simulink model "PSO_PID_Frecuencia"  (R2025a)
settings: Solver=FixedStepAuto  StartTime=0.0  StopTime=19  FixedStep=0.01  RelTol=1e-3
undefined symbols (not defined in the file or in its folder): CR, Kc_sim, LF, Td_sim, Ti_sim
libraries: instrumentseriallib x3
settings Model: Creator=jorge  LastModifiedBy=sergio2416

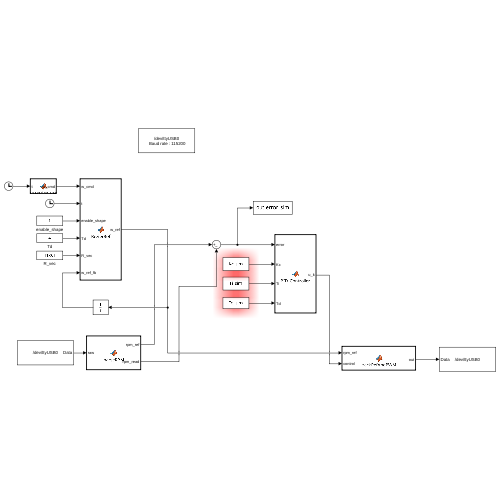
[thumbnail: Simulink's stored preview of the top-level diagram]
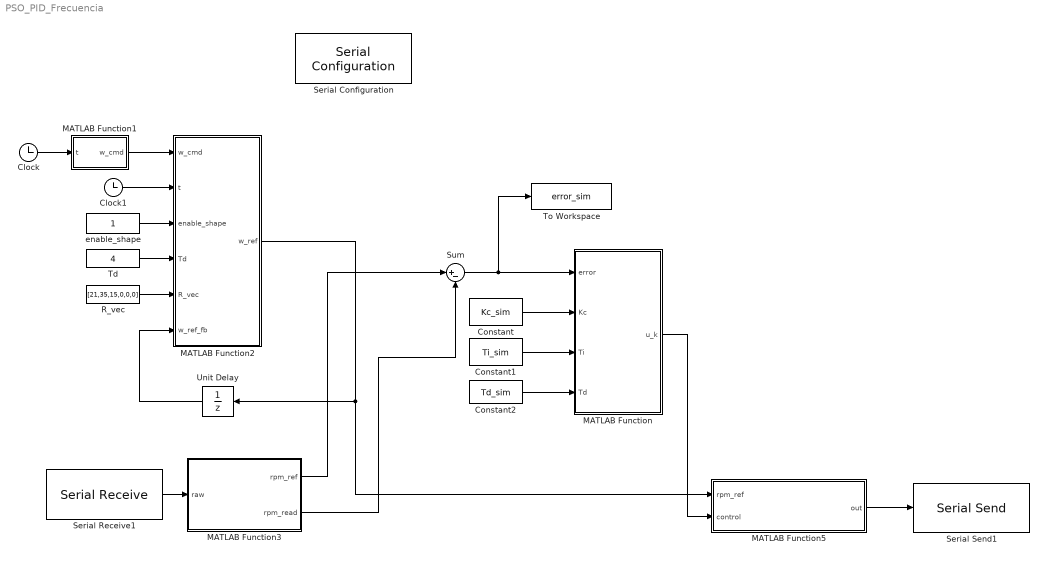
== system PSO_PID_Frecuencia ==
  Clock : Clock
  Clock1 : Clock
  Constant : Constant  Value=Kc_sim
  Constant1 : Constant  Value=Ti_sim
  Constant2 : Constant  Value=Td_sim
  MATLAB Function : MATLAB Function  TreatAsAtomicUnit=on
  MATLAB Function1 : MATLAB Function  TreatAsAtomicUnit=on
  MATLAB Function2 : MATLAB Function  TreatAsAtomicUnit=on
  MATLAB Function3 : MATLAB Function  TreatAsAtomicUnit=on
  MATLAB Function5 : MATLAB Function  TreatAsAtomicUnit=on
  R_vec : Constant  Value=[21,35,15,0,0,0]  SampleTime=-1
  Serial Configuration : instrumentseriallib/Serial Configuration  Priority=-200000  PortSel=/dev/ttyUSB0  Port=/dev/ttyUSB0  ComPort=/dev/ttyUSB0  BaudRate=115200  DataBits=8  Parity=none  StopBits=1  ByteOrder=little-endian  FlowControl=none  Timeout=10  SimulateUsing=Interpreted execution  BlockInModel=on  aMode=1
  Serial Receive1 : instrumentseriallib/Serial Receive  Priority=1  PortSel=/dev/ttyUSB0  Port=/dev/ttyUSB0  ComPort=/dev/ttyUSB0  DataType=int16  SaveDataType=uint8  ToggleHeader=off  Header=[]  ToggleDataSize=on  DataSize=[2 1]  ToggleTerminator=off  Terminator=CR/LF ('\r\n')  CustomTerminator=[]  InputFormat=Column major  EnableBlockingMode=on  ActionDataUnavailable=Output last received value  ActionWhenDataUnavailable=Output last received value  CustomValue=0  SampleTime=0.01  SimulateUsing=Interpreted execution  BlockInModel=on  aMode=1  LibraryInUse=instrumentlib
  Serial Send1 : instrumentseriallib/Serial Send  Priority=1  PortSel=/dev/ttyUSB0  Port=/dev/ttyUSB0  ComPort=/dev/ttyUSB0  Header=[]  Terminator=<none>  CustomTerminator=[]  EnableBlockingMode=off  SimulateUsing=Interpreted execution  BlockInModel=on  aMode=1
  Sum : Sum  Inputs=|+-
  Td : Constant  Value=4  SampleTime=-1
  To Workspace : ToWorkspace  VariableName=error_sim  SaveFormat=Timeseries  SampleTime=-1
  Unit Delay : UnitDelay  SampleTime=-1  HasFrameUpgradeWarning=on
  enable_shape : Constant  SampleTime=-1
  wires:
  Sum/1 -> To Workspace/1, MATLAB Function/1(error)
  Constant/1 -> MATLAB Function/2(Kc)
  Constant1/1 -> MATLAB Function/3(Ti)
  Constant2/1 -> MATLAB Function/4(Td)
  Clock/1 -> MATLAB Function1/1(t)
  Clock1/1 -> MATLAB Function2/2(t)
  enable_shape/1 -> MATLAB Function2/3(enable_shape)
  Td/1 -> MATLAB Function2/4(Td)
  MATLAB Function1/1(w_cmd) -> MATLAB Function2/1(w_cmd)
  R_vec/1 -> MATLAB Function2/5(R_vec)
  Unit Delay/1 -> MATLAB Function2/6(w_ref_fb)
  MATLAB Function5/1(out) -> Serial Send1/1
  Serial Receive1/1 -> MATLAB Function3/1(raw)
  MATLAB Function3/2(rpm_read) -> Sum/2
  MATLAB Function3/1(rpm_ref) -> Sum/1
  MATLAB Function2/1(w_ref) -> MATLAB Function5/1(rpm_ref), Unit Delay/1
  MATLAB Function/1(u_k) -> MATLAB Function5/2(control)

== matlab function PSO_PID_Frecuencia/MATLAB Function1 ==
  data: t input; w_cmd output
function w_cmd = Generador_Perfil(t)
    % Genera la señal escalón para alimentar al suavizador Bezier
    % Secuencia: 540 -> 1160 -> 800
    
    % --- CONFIGURACIÓN DE TIEMPOS ---
    % Td es 4 segundos. Dejamos un margen para que se estabilice.
    t_inicio = 1;   % Tiempo para el primer cambio (540 -> 1160)
    t_bajada = 10;  % Tiempo para el segundo cambio (1160 -> 800)
    
    % --- LÓGICA DE COMANDO ---
    if t < t_inicio
        % Estado inicial
        w_cmd = 600;
        
    elseif t >= t_inicio && t < t_bajada
        % Primer escalón: Subida
        w_cmd = 1160;
        
    else
        % Segundo escalón: Bajada
        w_cmd = 800;
    end
end

== matlab function PSO_PID_Frecuencia/MATLAB Function2 ==
  settings: updateMethod=DISCRETE
  data: w_cmd input; t input; w_ref output; enable_shape input; Td input; R_vec input; w_ref_fb input
function w_ref = BezierRef(w_cmd, t, enable_shape, Td, R_vec, w_ref_fb)
% =================================================================
% VERSIÓN 6 (Corrección de arranque en cero)
% =================================================================
%
% Entradas:
%   w_cmd     : setpoint deseado (de la GUI)
%   t         : tiempo absoluto (Clock)
%   enable_shape : 1 = perfilar, 0 = paso directo
%   Td        : duración de la transición [s]
%   R_vec     : [r1..r6] coeficientes del polinomio
%   w_ref_fb  : w_ref anterior (feedback vía Memory/Unit Delay)
%
% Salida:
%   w_ref     : referencia suavizada

% --- estados persistentes ---
persistent w0 wf t0 last_cmd is_initialized

% --- Lógica de inicialización en el primer paso de ejecución ---
if isempty(is_initialized) || t == 0 % Se reinicia si el tiempo es 0
    is_initialized = true; 
    
    % --- CORRECCIÓN AQUÍ ---
    % Antes decía: w0 = w_ref_fb; (Esto tomaba el 0 del Unit Delay)
    % Ahora dice:
    w0 = w_cmd;  % Forzamos a que el punto de partida sea el comando actual (540)
    wf = w_cmd;
    
    t0 = t;
    last_cmd = w_cmd;
end

% --- FIX 1: Detecta cambio de comando con tolerancia ---
if abs(w_cmd - last_cmd) > 1e-6
    % AQUÍ SÍ usamos w_ref_fb, porque queremos una curva suave desde
    % donde nos quedamos anteriormente.
    w0 = w_ref_fb;
    wf = w_cmd;
    t0 = t;
    last_cmd = w_cmd;
end

% Paso directo si está desactivado
if enable_shape == 0 || Td <= 0
    w_ref = w_cmd;
    w0 = w_cmd; 
    wf = w_cmd;
    last_cmd = w_cmd;
    return
end

% Progreso normalizado en [0,1]
s = (t - t0) / Td;

if s <= 0
    alpha = 0;
elseif s >= 1
    alpha = 1;
else
    % Bezier polinómico
    if numel(R_vec) < 6
        alpha = s; % Fallback a rampa lineal
    else
        r1 = R_vec(1); r2 = R_vec(2); r3 = R_vec(3);
        r4 = R_vec(4); r5 = R_vec(5); r6 = R_vec(6);
        
        % Validación de coeficientes
        if abs((r1 - r2 + r3 - r4 + r5 - r6) - 1.0) > 1e-3
            alpha = s^5;
        else
            alpha = (s.^5).*(r1 - r2*s + r3*s.^2 - r4*s.^3 + r5*s.^4 - r6*s.^5);
        end
    end
    
    % Clampeo por seguridad numérica
    if alpha < 0, alpha = 0; end
    if alpha > 1, alpha = 1; end
end

% Interpolación entre w0 y wf
w_ref = w0 + alpha*(wf - w0);
end

== matlab function PSO_PID_Frecuencia/MATLAB Function3 ==
  data: rpm_ref output; rpm_read output; raw input
function [rpm_ref, rpm_read] = parseRPM(raw)
%#codegen
% raw: 1x2 uint16 vector received from ESP32
% rpm_read: measured RPM from encoder
% rpm_ref:  reference RPM echoed back from ESP32

rpm_read = double(raw(2));   % first  uint16 from ESP32
rpm_ref  = double(raw(1));   % second uint16 from ESP32
end

== matlab function PSO_PID_Frecuencia/MATLAB Function5 ==
  data: rpm_ref input; control input; out output
function out = packRefAndPWM(rpm_ref, control)
% Esta función ahora empaqueta [rpm_ref, frequency_hz]
% El 'control_signal' (antes 'voltage') viene de 0-60 desde el "Knob".

% --- 1. Escalado lineal ---
% Frecuencia (0-60 Hz)
target_freq = control;

% --- 2. Empaquetado ---
% Convierte ambos valores a uint16 para enviar por UART
freq_u16 = uint16(target_freq);
rpm_ref_u16 = uint16(rpm_ref);

% El ESP32 espera recibir: [rpm_ref, frecuencia_en_hz]
out = uint16([rpm_ref_u16, freq_u16]);

end

== matlab function PSO_PID_Frecuencia/MATLAB Function ==
  data: error input; u_k output; Kc input; Ti input; Td input
function u_k = PID_Controller(error, Kc, Ti, Td)
    % ENTRADAS (Puertos en Simulink):
    %   error: Señal de error (Referencia - Salida)
    %   Kc, Ti, Td: Parámetros que vienen del Workspace (vía bloques Constant)
    
    % PARÁMETROS FIJOS (Ajusta si tu muestreo es distinto)
    Ts_s = 0.01;  % Tiempo de muestreo
    N = 100;      % Coeficiente del filtro derivativo

    % VARIABLES DE ESTADO (Persistentes)
    persistent error_prev integral_prev derivative_prev

    % INICIALIZACIÓN (Se ejecuta al inicio de CADA simulación 'sim')
    if isempty(error_prev)
        error_prev = 0.0;
        integral_prev = 0.0; % Ojo: Si tu salida debe empezar en 20, considera inicializar esto distinto
        derivative_prev = 0.0;
    end

    % --- 1. Proporcional ---
    p_k = Kc * error;

    % --- 2. Integral ---
    % Protección para Ti muy pequeño
    if Ti < 1e-6
        i_k = 0;
    else
        % Integración Euler
        i_k = integral_prev + (Kc * Ts_s / Ti) * error;
    end

    % --- 3. Derivativo ---
    c1 = 1.0 / (1.0 + Ts_s * N);
    c2 = (Kc * Td * N) / (1.0 + Ts_s * N);
    d_k = c1 * derivative_prev + c2 * (error - error_prev);

    % --- 4. Salida Total ---
    u_k_total = p_k + i_k + d_k;

    % --- 5. Saturación [20 a 50] ---
    u_k_saturado = u_k_total;
    
    if u_k_saturado > 50.0
        u_k_saturado = 50.0;
    elseif u_k_saturado < 20.0
        u_k_saturado = 20.0;
    end

    % --- 6. Actualización de Estados (Anti-Windup) ---
    % Si la salida NO se saturó, actualizamos la integral.
    % Si SE saturó, mantenemos la integral anterior (congelamos).
    if u_k_total == u_k_saturado
        integral_prev = i_k;
    end
    
    derivative_prev = d_k;
    error_prev = error;

    % Salida final
    u_k = u_k_saturado;
end
